simulink model "Moving_Average_sim"  (R2025a)
settings: Solver=VariableStepAuto  StartTime=0.0  StopTime=20  RelTol=1e-3
libraries: simulink x1
settings Model: Creator=Luiz  LastModifiedBy=Luiz
settings OptimizationCC: BlockReduction=off  ConditionallyExecuteInputs=off  DefaultParameterBehavior=Inlined
settings DebuggingCC: AlgebraicLoopMsg=error  SingleTaskRateTransMsg=error
settings HardwareCC: ProdBitPerPointer=32.0  ProdBitPerSizeT=32.0  ProdBitPerPtrDiffT=32.0  ProdLargestAtomicFloat=None  ProdIntDivRoundTo=Undefined  ProdEndianess=Unspecified  ProdWordSize=32.0  ProdHWDeviceType=ASIC/FPGA->ASIC/FPGA  TargetBitPerPointer=64.0  TargetBitPerSizeT=64.0  TargetBitPerPtrDiffT=64.0  TargetLongLongMode=on  TargetIntDivRoundTo=Zero  TargetEndianess=LittleEndian  TargetWordSize=64.0  TargetHWDeviceType=Custom Processor->MATLAB Host Computer  ProdEqTarget=off

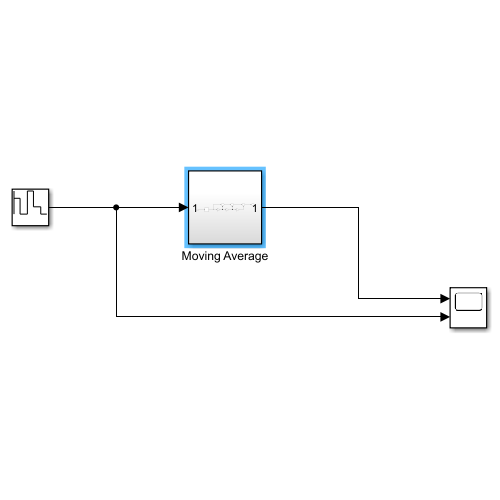
[thumbnail: Simulink's stored preview of the top-level diagram]
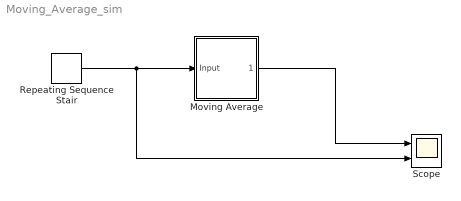
== system Moving_Average_sim ==
  Moving Average : Subsystem
  Repeating Sequence Stair : simulink/Sources/Repeating Sequence Stair  OutValues=[3 1 4 2 1].'  tsamp=-1  OutMin=[]  OutMax=[]  OutDataTypeStr=double  OutputDataTypeScalingMode=double  OutDataType=fixdt(0,8)  ConRadixGroup=Best Precision: Vector-wise  OutScaling=2^-12
      settings: LibrarySourceBlock=|
      | hdlsllib/Sources/Repeating
      | Sequence
      | Stair
  Scope : Scope  NumInputPorts=2
      settings: ActiveDisplayYMinimum=-38.789014690197241  ActiveDisplayYMaximum=12.26224780980278  DataLoggingVariableName=ScopeData2  DataLoggingSaveFormat=Array
  wires:
  Repeating Sequence Stair/1 -> Scope/2, Moving Average/1(Input)
  Moving Average/1(Output) -> Scope/1

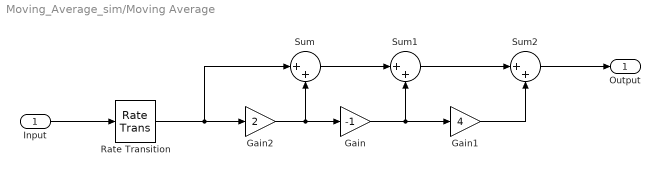
== system Moving_Average_sim/Moving Average ==
  Input : Inport  OutDataTypeStr=double  SampleTime=0.0001
  Gain : Gain  Gain=-1  OutDataTypeStr=double
  Gain1 : Gain  Gain=4  OutDataTypeStr=double
  Gain2 : Gain  Gain=2  OutDataTypeStr=double
  Rate Transition : RateTransition
  Sum : Sum  Inputs=|++
  Sum1 : Sum  Inputs=|++
  Sum2 : Sum  Inputs=|++
  Output : Outport  OutDataTypeStr=double  SampleTime=0.0001  VectorParamsAs1DForOutWhenUnconnected=off
  wires:
  Sum2/1 -> Output/1
  Gain1/1 -> Sum2/2
  Sum1/1 -> Sum2/1
  Sum/1 -> Sum1/1
  Gain2/1 -> Gain/1, Sum/2
  Gain/1 -> Gain1/1, Sum1/2
  Input/1 -> Rate Transition/1
  Rate Transition/1 -> Sum/1, Gain2/1
